simulink library "lib_fuel_converter"  (Simulink 7.9)
settings: Solver=ode45  SolverMode=SingleTasking  StartTime=0.0  StopTime=10.0  RelTol=1e-3
undefined symbols (not defined in the file or in its folder): acc_mech_eff, acc_mech_pwr, acc_mech_trq, air_cp, amb_tmp, cyc_mph, ex_gas_cp, fc_acc_mass, fc_base_mass, fc_c2i_th_cond, fc_c_init_tmp, fc_cl2h_eff, fc_CO2_to_FUELgps, fc_co_map, fc_co_map_c2h, fc_cold, fc_cold_tmp, fc_cp, fc_ct_trq, fc_eff_scale, fc_emisv, fc_exflow_map, fc_ext_sarea, fc_extmp_map, fc_fuel_den, fc_fuel_lhv, fc_fuel_map, fc_fuel_map_c2h, fc_h2x_th_cond, fc_h_air_flow, fc_h_cp, fc_h_init_tmp, fc_hc_map, fc_hc_map_c2h, fc_hood_emisv, fc_hood_sarea, fc_i2x_th_cond, fc_i_init_tmp, fc_inertia, fc_map_spd, fc_map_trq, fc_max_trq, fc_nn_model_name, fc_nox_map, fc_nox_map_c2h, fc_o2_map, fc_pm_map, fc_pm_map_c2h, fc_pwr_scale, fc_spd_scale, fc_trq_scale, fc_tstat, fc_x_init_tmp, fd_ratio, gb_num_init, gb_ratio, pow, vc_idle_spd, vc_key_on, veh_glider_mass ... (+2)
libraries: lib_fuel_converter x6, lib_etc x4
(part 2 of 4)

== system lib_fuel_converter/fuel converter  <fc> for series/spinning up or spinning down ==
  spd command (rad/s) : Inport
  engine disconnected from drivetrain : Inport  Port=2
  previous engine spd (rad/s) : Inport  Port=3
  Constant : Constant  Value=0
  Constant1 : Constant  Value=vc_idle_spd
  MinMax : MinMax  Inputs=2  SaturateOnIntegerOverflow=on  InputSameDT=on
  MinMax1 : MinMax  Function=max  Inputs=2  SaturateOnIntegerOverflow=on  InputSameDT=on
  Mux3 : Mux  Inputs=3
  Product : Product  SaturateOnIntegerOverflow=on  RndMeth=Zero  InputSameDT=on  OutDataTypeStr=Inherit: Same as first input
  Product2 : Product  SaturateOnIntegerOverflow=on  RndMeth=Zero  InputSameDT=on  OutDataTypeStr=Inherit: Same as first input
  Relational Operator : RelationalOperator  Operator=<=  InputSameDT=on
  Sum : Sum  Inputs=|++  SaturateOnIntegerOverflow=on  InputSameDT=on  OutDataTypeStr=Inherit: Same as first input
  Sum1 : Sum  Inputs=|+-  SaturateOnIntegerOverflow=on  InputSameDT=on  OutDataTypeStr=Inherit: Same as first input
  Sum2 : Sum  SaturateOnIntegerOverflow=on  InputSameDT=on  OutDataTypeStr=Inherit: Same as first input
  Switch: map torque : Switch  Threshold=eps  SaturateOnIntegerOverflow=on  InputSameDT=on
  T_closed throttle : Subsystem
  T_max : Subsystem
  alpha : Gain  Gain=1/(fc_inertia+eps)  SaturateOnIntegerOverflow=on  OutDataTypeStr=Inherit: Same as input  ParamDataTypeStr=Inherit: Same as input
  dt : Subsystem
  effect of inertia (Nm) : Subsystem
  just started spin-down/spin-up : Subsystem
  no-lag Reset Integrator : Subsystem  mask(No-lag Reset Integrator){initval=vc_idle_spd}
      mask prompts: initval "Initial Value"
      mask help: No-lag Reset Integrator
      mask Help: Integrates first input using Euler technique.\nAt the time step that input 2 <> zero,\noutput is reset to input 3.
      mask Display: disp('1/s\nw/ reset\nno lag')
  map trq (Nm) spd (rad/s) trq to drivetrain (Nm) : Outport  InitialOutput=0
  wires:
  T_max/1(T_max) -> MinMax/1
  MinMax/1 -> Switch: map torque/1
  T_closed throttle/1(T_closed throttle) -> Switch: map torque/3
  Switch: map torque/1 -> Mux3/1, Sum1/1
  Relational Operator/1 -> Switch: map torque/2
  alpha/1 -> Product/1, no-lag Reset Integrator/1(in_1)
  previous engine spd (rad/s)/1 -> T_closed throttle/1(w_APU), T_max/1(w_APU), effect of inertia (Nm)/2(prev spd), Relational Operator/1, Sum2/2
  spd command (rad/s)/1 -> Relational Operator/2, effect of inertia (Nm)/1(req'd spd (rad/s))
  no-lag Reset Integrator/1(out_1) -> MinMax1/1
  just started spin-down/spin-up/1(trigger) -> no-lag Reset Integrator/2(in_2)
  Sum2/1 -> no-lag Reset Integrator/3(in_3)
  engine disconnected from drivetrain/1 -> just started spin-down/spin-up/1(state)
  Product/1 -> Sum2/1
  dt/1(out_1) -> Product/2
  Mux3/1 -> map trq (Nm) spd (rad/s) trq to drivetrain (Nm)/1
  Constant/1 -> Mux3/3
  Constant1/1 -> Product2/1
  [engine_on] -> Product2/2
  Product2/1 -> MinMax1/2
  MinMax1/1 -> Mux3/2
  effect of inertia (Nm)/1((Nm)) -> Sum/1
  Sum/1 -> MinMax/2
  [acc_mech_trq_est] -> Sum/2
  Sum1/1 -> alpha/1
  [acc_mech_trq_est] -> Sum1/2

== system lib_fuel_converter/fuel converter  <fc> prius/Block NOTES ==
  note: This block models the internal combustion engine, and includes inertia effects,
      | performance limits, accessory loads, and temperature transient effects on fuel
      | use, engine-out emissions, and catalyst efficiency.  There are 'leads' to the
      | engine controller here, which controller determines whether the engine is on.

== system lib_fuel_converter/fuel converter  <fc> prius/fuel use and EO emis Configurable Subsystem ==
  T (Nm) : Inport
  w (rad/s) : Inport  Port=2
  fuel use and EO emis : lib_fuel_converter/configurable subsystems/fuel use and EO emis
      settings: RTWFcnNameOpts=Auto  RTWFileNameOpts=Auto
  cumulative fuel  use (gal) : Outport
  "FC ON?, EOem, MFex, Tex, O2ex" : Outport  Port=2
  Vv,Tfc : Outport  Port=3
  wires:
  T (Nm)/1 -> fuel use and EO emis/1
  w (rad/s)/1 -> fuel use and EO emis/2
  fuel use and EO emis/1 -> cumulative fuel  use (gal)/1
  fuel use and EO emis/2 -> "FC ON?, EOem, MFex, Tex, O2ex"/1
  fuel use and EO emis/3 -> Vv,Tfc/1

== system lib_fuel_converter/fuel converter  <fc> prius/providing trq (+ive or -ive) ==
  req'd trq (Nm) : Inport
  req'd spd (rad/s) : Inport  Port=2
  prev engine spd (rad/s) : Inport  Port=3
  Mux3 : Mux
  Product : Product  SaturateOnIntegerOverflow=on  RndMeth=Zero  InputSameDT=on  OutDataTypeStr=Inherit: Same as first input
  Sum1 : Sum  Inputs=+--  SaturateOnIntegerOverflow=on  InputSameDT=on  OutDataTypeStr=Inherit: Same as first input
  Sum2 : Sum  Inputs=+++  SaturateOnIntegerOverflow=on  InputSameDT=on  OutDataTypeStr=Inherit: Same as first input
  accessories (Nm) : Subsystem
  effect of inertia (Nm) : Subsystem
  enforce engine limits : Subsystem
  map trq (Nm) spd (rad/s) trq to drivetrain (Nm) accessory load (W) : Outport  InitialOutput=0
  tag scope: engine_rpm=global
  wires:
  req'd spd (rad/s)/1 -> Product/2, enforce engine limits/2(req'd engine spd (rad/s))
  Product/1 -> Mux3/4
  Sum1/1 -> Mux3/3
  Mux3/1 -> map trq (Nm) spd (rad/s) trq to drivetrain (Nm) accessory load (W)/1
  prev engine spd (rad/s)/1 -> effect of inertia (Nm)/2(prev spd)
  enforce engine limits/1(limited engine brake trq (Nm)) -> Mux3/1, Sum1/1
  enforce engine limits/2(limited engine spd (rad/s)) -> effect of inertia (Nm)/1(req'd spd (rad/s)), accessories (Nm)/1(w_APU), Mux3/2, [engine_rpm]
  req'd trq (Nm)/1 -> Sum2/1
  effect of inertia (Nm)/1((Nm)) -> Sum1/2, Sum2/2
  accessories (Nm)/1(T_acc) -> Product/1, Sum1/3, Sum2/3
  Sum2/1 -> enforce engine limits/1(req'd engine trq (Nm))

== system lib_fuel_converter/configurable subsystems/fuel use and EO emis/Block NOTES ==
  note: This block determines actual fuel use and engine-out emissions
      | given the fully hot values and the engine coolant temperature.
      | The correlations used here were developed at NREL using
      | FTP data collected under subcontract by JDM & Associates.
      | Note: PM hot/cold relation assumed same as HC

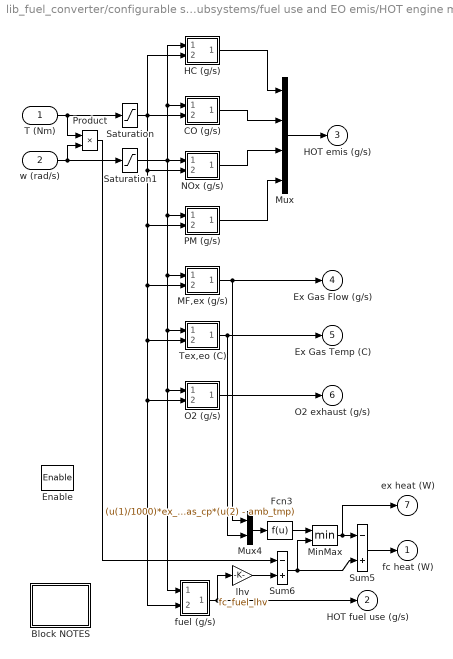
== system lib_fuel_converter/configurable subsystems/fuel use and EO emis/HOT engine maps  ==
  T (Nm) : Inport
  w (rad/s) : Inport  Port=2
  Enable : EnablePort  StatesWhenEnabling=reset
  Block NOTES : Subsystem
      mask Display: disp('Block\nNOTES')
  CO (g/s) : Subsystem  mask(2-D Table Lookup){xindex=fc_map_spd*fc_spd_scale, yindex=fc_map_trq*fc_trq_scale, table=fc_co_map*fc_spd_scale*fc_trq_scale}
      mask prompts: xindex "X Index"; yindex "Y Index"
      mask help:
      | Two Dimensional Table Lookup
      | The first input corresponds to X Index and the second input corresponds to the Y Index
      mask init:
      | sftab2chk(xindex,yindex,table);
      mask Help: This block returns a linearly interpolated intersection from the table using the X index (which corresponds to the rows of the table) and the Y index (which corresponds to the columns of the table).  Extrapolation is used.
      mask Display: plot(-10,-10,110,110,[90,50,10],[90,40,30],[90,50,10],[50,26,20],[90,50,10],[22,13,10])
  Fcn3 : Fcn  Expr=(u(1)/1000)*ex_gas_cp*(u(2) - amb_tmp)
  HC (g/s) : Subsystem  mask(2-D Table Lookup){xindex=fc_map_spd*fc_spd_scale, yindex=fc_map_trq*fc_trq_scale, table=fc_hc_map*fc_spd_scale*fc_trq_scale}
      mask prompts: xindex "X Index"; yindex "Y Index"
      mask help:
      | Two Dimensional Table Lookup
      | The first input corresponds to X Index and the second input corresponds to the Y Index
      mask init:
      | sftab2chk(xindex,yindex,table);
      mask Help: This block returns a linearly interpolated intersection from the table using the X index (which corresponds to the rows of the table) and the Y index (which corresponds to the columns of the table).  Extrapolation is used.
      mask Display: plot(-10,-10,110,110,[90,50,10],[90,40,30],[90,50,10],[50,26,20],[90,50,10],[22,13,10])
  MF,ex (g/s) : Subsystem  mask(2-D Table Lookup){xindex=fc_map_spd*fc_spd_scale, yindex=fc_map_trq*fc_trq_scale, table=fc_exflow_map*fc_spd_scale*fc_trq_scale}
      mask prompts: xindex "X Index"; yindex "Y Index"
      mask help:
      | Two Dimensional Table Lookup
      | The first input corresponds to X Index and the second input corresponds to the Y Index
      mask init:
      | sftab2chk(xindex,yindex,table);
      mask Help: This block returns a linearly interpolated intersection from the table using the X index (which corresponds to the rows of the table) and the Y index (which corresponds to the columns of the table).  Extrapolation is used.
      mask Display: plot(-10,-10,110,110,[90,50,10],[90,40,30],[90,50,10],[50,26,20],[90,50,10],[22,13,10])
  MinMax : MinMax  Inputs=2  SaturateOnIntegerOverflow=on  InputSameDT=on
  Mux : Mux
  Mux4 : Mux  Inputs=2
  NOx (g/s) : Subsystem  mask(2-D Table Lookup){xindex=fc_map_spd*fc_spd_scale, yindex=fc_map_trq*fc_trq_scale, table=fc_nox_map*fc_spd_scale*fc_trq_scale}
      mask prompts: xindex "X Index"; yindex "Y Index"
      mask help:
      | Two Dimensional Table Lookup
      | The first input corresponds to X Index and the second input corresponds to the Y Index
      mask init:
      | sftab2chk(xindex,yindex,table);
      mask Help: This block returns a linearly interpolated intersection from the table using the X index (which corresponds to the rows of the table) and the Y index (which corresponds to the columns of the table).  Extrapolation is used.
      mask Display: plot(-10,-10,110,110,[90,50,10],[90,40,30],[90,50,10],[50,26,20],[90,50,10],[22,13,10])
  O2 (g/s) : Subsystem  mask(2-D Table Lookup){xindex=fc_map_spd*fc_spd_scale, yindex=fc_map_trq*fc_trq_scale, table=fc_o2_map*fc_spd_scale*fc_trq_scale}
      mask prompts: xindex "X Index"; yindex "Y Index"
      mask help:
      | Two Dimensional Table Lookup
      | The first input corresponds to X Index and the second input corresponds to the Y Index
      mask init:
      | sftab2chk(xindex,yindex,table);
      mask Help: This block returns a linearly interpolated intersection from the table using the X index (which corresponds to the rows of the table) and the Y index (which corresponds to the columns of the table).  Extrapolation is used.
      mask Display: plot(-10,-10,110,110,[90,50,10],[90,40,30],[90,50,10],[50,26,20],[90,50,10],[22,13,10])
  PM (g/s) : Subsystem  mask(2-D Table Lookup){xindex=fc_map_spd*fc_spd_scale, yindex=fc_map_trq*fc_trq_scale, table=fc_pm_map*fc_spd_scale*fc_trq_scale}
      mask prompts: xindex "X Index"; yindex "Y Index"
      mask help:
      | Two Dimensional Table Lookup
      | The first input corresponds to X Index and the second input corresponds to the Y Index
      mask init:
      | sftab2chk(xindex,yindex,table);
      mask Help: This block returns a linearly interpolated intersection from the table using the X index (which corresponds to the rows of the table) and the Y index (which corresponds to the columns of the table).  Extrapolation is used.
      mask Display: plot(-10,-10,110,110,[90,50,10],[90,40,30],[90,50,10],[50,26,20],[90,50,10],[22,13,10])
  Product : Product  SaturateOnIntegerOverflow=on  RndMeth=Zero  InputSameDT=on  OutDataTypeStr=Inherit: Same as first input
  Saturation : Saturate  UpperLimit=max(fc_map_trq*fc_trq_scale)  LowerLimit=min(fc_map_trq*fc_trq_scale)
  Saturation1 : Saturate  UpperLimit=max(fc_map_spd*fc_spd_scale)  LowerLimit=min(fc_map_spd*fc_spd_scale)
  Sum5 : Sum  Inputs=-+  SaturateOnIntegerOverflow=on  InputSameDT=on  OutDataTypeStr=Inherit: Same as first input
  Sum6 : Sum  Inputs=-+  SaturateOnIntegerOverflow=on  InputSameDT=on  OutDataTypeStr=Inherit: Same as first input
  Tex,eo (C) : Subsystem  mask(2-D Table Lookup){xindex=fc_map_spd*fc_spd_scale, yindex=fc_map_trq*fc_trq_scale, table=fc_extmp_map}
      mask prompts: xindex "X Index"; yindex "Y Index"
      mask help:
      | Two Dimensional Table Lookup
      | The first input corresponds to X Index and the second input corresponds to the Y Index
      mask init:
      | sftab2chk(xindex,yindex,table);
      mask Help: This block returns a linearly interpolated intersection from the table using the X index (which corresponds to the rows of the table) and the Y index (which corresponds to the columns of the table).  Extrapolation is used.
      mask Display: plot(-10,-10,110,110,[90,50,10],[90,40,30],[90,50,10],[50,26,20],[90,50,10],[22,13,10])
  fuel (g/s) : Subsystem  mask(2-D Table Lookup){xindex=fc_map_spd*fc_spd_scale, yindex=fc_map_trq*fc_trq_scale, table=fc_fuel_map*fc_spd_scale*fc_trq_scale/fc_eff_scale}
      mask prompts: xindex "X Index"; yindex "Y Index"
      mask help:
      | Two Dimensional Table Lookup
      | The first input corresponds to X Index and the second input corresponds to the Y Index
      mask init:
      | sftab2chk(xindex,yindex,table);
      mask Help: This block returns a linearly interpolated intersection from the table using the X index (which corresponds to the rows of the table) and the Y index (which corresponds to the columns of the table).  Extrapolation is used.
      mask Display: plot(-10,-10,110,110,[90,50,10],[90,40,30],[90,50,10],[50,26,20],[90,50,10],[22,13,10])
  lhv : Gain  Gain=fc_fuel_lhv  SaturateOnIntegerOverflow=on  OutDataTypeStr=Inherit: Same as input  ParamDataTypeStr=Inherit: Same as input
  fc heat (W) : Outport  OutputWhenDisabled=reset  InitialOutput=eps
  HOT fuel use (g/s) : Outport  Port=2  OutputWhenDisabled=reset  InitialOutput=eps
  HOT emis (g/s) : Outport  Port=3  OutputWhenDisabled=reset  InitialOutput=eps
  Ex Gas Flow (g/s) : Outport  Port=4  OutputWhenDisabled=reset  InitialOutput=eps
  Ex Gas Temp (C) : Outport  Port=5  OutputWhenDisabled=reset  InitialOutput=amb_tmp
  O2 exhaust (g/s) : Outport  Port=6  OutputWhenDisabled=reset  InitialOutput=0
  ex heat (W) : Outport  Port=7  OutputWhenDisabled=reset  InitialOutput=eps
  wires:
  PM (g/s)/1(table out) -> Mux/4
  HC (g/s)/1(table out) -> Mux/1
  CO (g/s)/1(table out) -> Mux/2
  NOx (g/s)/1(table out) -> Mux/3
  Mux/1 -> HOT emis (g/s)/1
  MF,ex (g/s)/1(table out) -> Ex Gas Flow (g/s)/1, Mux4/1
  Tex,eo (C)/1(table out) -> Ex Gas Temp (C)/1, Mux4/2
  Saturation1/1 -> NOx (g/s)/1(x0), MF,ex (g/s)/1(x0), Tex,eo (C)/1(x0), fuel (g/s)/1(x0), O2 (g/s)/1(x0), PM (g/s)/1(x0), CO (g/s)/1(x0), HC (g/s)/1(x0)
  Saturation/1 -> CO (g/s)/2(y0), MF,ex (g/s)/2(y0), Tex,eo (C)/2(y0), fuel (g/s)/2(y0), O2 (g/s)/2(y0), PM (g/s)/2(y0), NOx (g/s)/2(y0), HC (g/s)/2(y0)
  T (Nm)/1 -> Saturation/1, Product/1
  w (rad/s)/1 -> Saturation1/1, Product/2
  Mux4/1 -> Fcn3/1
  Sum5/1 -> fc heat (W)/1
  Fcn3/1 -> MinMax/1
  MinMax/1 -> Sum5/1, ex heat (W)/1
  Sum6/1 -> Sum5/2, MinMax/2
  Product/1 -> Sum6/1
  fuel (g/s)/1(table out) -> HOT fuel use (g/s)/1, lhv/1
  lhv/1 -> Sum6/2
  O2 (g/s)/1(table out) -> O2 exhaust (g/s)/1

== system lib_fuel_converter/configurable subsystems/fuel use and EO emis/fc temp ==
  note: h
  note: x
  note: i
  note: c
  veh spd (m/s) : Inport
  key ON? : Inport  Port=2
  fc ON? : Inport  Port=3
  Qfc (W) : Inport  Port=4
  "1/ " : Gain  Gain=1/(0.2*fc_base_mass*fc_pwr_scale*fc_cp)  SaturateOnIntegerOverflow=on  OutDataTypeStr=Inherit: Same as input  ParamDataTypeStr=Inherit: Same as input
  1/Ci : Gain  Gain=1/(0.8*fc_base_mass*fc_pwr_scale*fc_cp)  SaturateOnIntegerOverflow=on  OutDataTypeStr=Inherit: Same as input  ParamDataTypeStr=Inherit: Same as input
  1/Cx : Gain  Gain=1/(fc_acc_mass*fc_pwr_scale*fc_cp)  SaturateOnIntegerOverflow=on  OutDataTypeStr=Inherit: Same as input  ParamDataTypeStr=Inherit: Same as input
  1/mcp : Gain  Gain=1/(0.1*veh_glider_mass*fc_pwr_scale*fc_h_cp)  SaturateOnIntegerOverflow=on  OutDataTypeStr=Inherit: Same as input  ParamDataTypeStr=Inherit: Same as input
  Block NOTES : Subsystem
      mask Display: disp('Block\nNOTES')
  Memory : Memory  X0=fc_h_init_tmp
  Mux3 : Mux
  Mux4 : Mux  Inputs=2
  Qc : Sum  SaturateOnIntegerOverflow=on  InputSameDT=on  OutDataTypeStr=Inherit: Same as first input
  Qc1 : Sum  Inputs=--+  SaturateOnIntegerOverflow=on  InputSameDT=on  OutDataTypeStr=Inherit: Same as first input
  Tcm : Integrator  InitialCondition=fc_c_init_tmp
  Tcx : Integrator  InitialCondition=fc_x_init_tmp
  Tcx1 : Integrator  InitialCondition=fc_i_init_tmp
  Tm : Integrator  InitialCondition=fc_h_init_tmp
  fc coolant : Subsystem  TreatAsAtomicUnit=on
  fc mass heat flow : Subsystem
  old fc coolant  temp. (C) : Subsystem
  Tfc_old  (C) : Outport  InitialOutput=0
  Qfc r,h : Outport  Port=2  InitialOutput=0
  Tfc  (C) : Outport  Port=3  InitialOutput=0
  tag scope: fc_hood_temp=global
  wires:
  Qc/1 -> "1/ "/1
  "1/ "/1 -> Tcm/1
  Qfc (W)/1 -> Qc/1
  fc mass heat flow/1(Qfc_c) -> Qc/2
  Qc1/1 -> 1/Ci/1
  1/Ci/1 -> Tcx1/1
  Tcm/1 -> Mux3/1
  fc mass heat flow/2(Qfc_i) -> Qc1/3, fc coolant/2("Qfc_i ")
  fc coolant/2(Qfc_htr) -> Qc1/2, Mux4/2
  fc coolant/1(Qfc_rad) -> Qc1/1, Mux4/1
  Tcx1/1 -> fc coolant/1(Tcl), Mux3/2
  Mux4/1 -> Qfc r,h/1
  1/Cx/1 -> Tcx/1
  fc mass heat flow/3(Qfc_x) -> 1/Cx/1
  key ON?/1 -> fc coolant/Enable
  Tcx/1 -> Mux3/3
  Tm/1 -> Mux3/4, Memory/1
  1/mcp/1 -> Tm/1
  fc mass heat flow/4(Qfc_h) -> 1/mcp/1
  Mux3/1 -> fc mass heat flow/2(fc_temp), Tfc  (C)/1
  old fc coolant  temp. (C)/1(fc coolant  temp (C)) -> Tfc_old  (C)/1
  veh spd (m/s)/1 -> old fc coolant  temp. (C)/2(veh spd), fc mass heat flow/1(veh spd)
  fc ON?/1 -> old fc coolant  temp. (C)/1(fc on?)
  Memory/1 -> [fc_hood_temp]

== system lib_fuel_converter/configurable subsystems/fuel use and EO emis/fc temp correct ==
  Coolant T (C) : Inport
  HOT fuel use (g/s) : Inport  Port=2
  HOT emis (g/s) : Inport  Port=3
  T (Nm) : Inport  Port=4
  w (rad/s) : Inport  Port=5
  Enable : EnablePort  StatesWhenEnabling=reset
  =1: use map based =0: use constant equation based : Constant  Value=fc_cold
  Switch : Switch  Threshold=eps  SaturateOnIntegerOverflow=on  InputSameDT=on
  Switch1 : Switch  Threshold=eps  SaturateOnIntegerOverflow=on  InputSameDT=on
  fc temp correct Constant Correction Factors (Equation Based) : Subsystem  TreatAsAtomicUnit=on
  fc temp correct Variable Correction Factors (Map Based) : Subsystem  TreatAsAtomicUnit=on
  fc_cold=0 : Logic  Operator=NOT
  fuel use (g/s) : Outport  OutputWhenDisabled=reset  InitialOutput=0
  EO emis (g/s) : Outport  Port=2  OutputWhenDisabled=reset  InitialOutput=0
  wires:
  =1: use map based =0: use constant equation based/1 -> fc_cold=0/1, fc temp correct Variable Correction Factors (Map Based)/Enable
  Coolant T (C)/1 -> fc temp correct Constant Correction Factors (Equation Based)/1(Coolant T (C)), fc temp correct Variable Correction Factors (Map Based)/1(Coolant T (C))
  HOT fuel use (g/s)/1 -> fc temp correct Constant Correction Factors (Equation Based)/2(HOT fuel use (g/s)), fc temp correct Variable Correction Factors (Map Based)/2(HOT fuel use (g/s))
  HOT emis (g/s)/1 -> fc temp correct Constant Correction Factors (Equation Based)/3(HOT emis (g/s)), fc temp correct Variable Correction Factors (Map Based)/3(HOT emis (g/s))
  fc temp correct Constant Correction Factors (Equation Based)/1(fuel use (g/s)) -> Switch/1
  fc_cold=0/1 -> fc temp correct Constant Correction Factors (Equation Based)/Enable, Switch/2, Switch1/2
  fc temp correct Variable Correction Factors (Map Based)/1(fuel use (g/s)) -> Switch/3
  fc temp correct Constant Correction Factors (Equation Based)/2(EO emis (g/s)) -> Switch1/1
  fc temp correct Variable Correction Factors (Map Based)/2(EO emis (g/s)) -> Switch1/3
  Switch/1 -> fuel use (g/s)/1
  Switch1/1 -> EO emis (g/s)/1
  T (Nm)/1 -> fc temp correct Variable Correction Factors (Map Based)/4(T (Nm))
  w (rad/s)/1 -> fc temp correct Variable Correction Factors (Map Based)/5(w (rad/s))

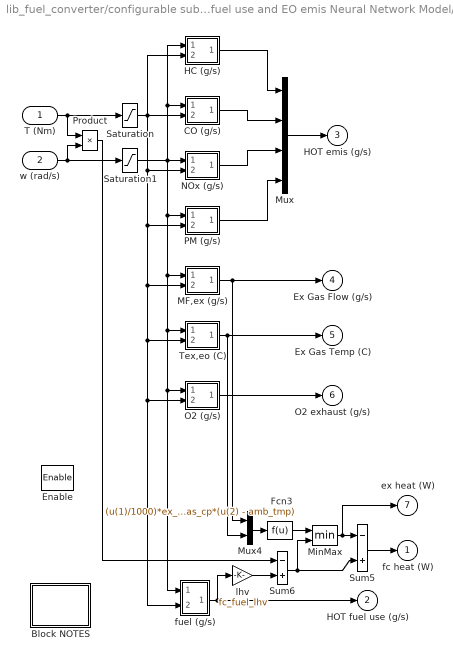
== system lib_fuel_converter/configurable subsystems/fuel use and EO emis Neural Network Model/HOT engine maps  ==
  T (Nm) : Inport
  w (rad/s) : Inport  Port=2
  Enable : EnablePort  StatesWhenEnabling=reset
  Block NOTES : Subsystem
      mask Display: disp('Block\nNOTES')
  CO (g/s) : Subsystem  mask(2-D Table Lookup){xindex=fc_map_spd*fc_spd_scale, yindex=fc_map_trq*fc_trq_scale, table=fc_co_map*fc_spd_scale*fc_trq_scale}
      mask prompts: xindex "X Index"; yindex "Y Index"
      mask help:
      | Two Dimensional Table Lookup
      | The first input corresponds to X Index and the second input corresponds to the Y Index
      mask init:
      | sftab2chk(xindex,yindex,table);
      mask Help: This block returns a linearly interpolated intersection from the table using the X index (which corresponds to the rows of the table) and the Y index (which corresponds to the columns of the table).  Extrapolation is used.
      mask Display: plot(-10,-10,110,110,[90,50,10],[90,40,30],[90,50,10],[50,26,20],[90,50,10],[22,13,10])
  Fcn3 : Fcn  Expr=(u(1)/1000)*ex_gas_cp*(u(2) - amb_tmp)
  HC (g/s) : Subsystem  mask(2-D Table Lookup){xindex=fc_map_spd*fc_spd_scale, yindex=fc_map_trq*fc_trq_scale, table=fc_hc_map*fc_spd_scale*fc_trq_scale}
      mask prompts: xindex "X Index"; yindex "Y Index"
      mask help:
      | Two Dimensional Table Lookup
      | The first input corresponds to X Index and the second input corresponds to the Y Index
      mask init:
      | sftab2chk(xindex,yindex,table);
      mask Help: This block returns a linearly interpolated intersection from the table using the X index (which corresponds to the rows of the table) and the Y index (which corresponds to the columns of the table).  Extrapolation is used.
      mask Display: plot(-10,-10,110,110,[90,50,10],[90,40,30],[90,50,10],[50,26,20],[90,50,10],[22,13,10])
  MF,ex (g/s) : Subsystem  mask(2-D Table Lookup){xindex=fc_map_spd*fc_spd_scale, yindex=fc_map_trq*fc_trq_scale, table=fc_exflow_map*fc_spd_scale*fc_trq_scale}
      mask prompts: xindex "X Index"; yindex "Y Index"
      mask help:
      | Two Dimensional Table Lookup
      | The first input corresponds to X Index and the second input corresponds to the Y Index
      mask init:
      | sftab2chk(xindex,yindex,table);
      mask Help: This block returns a linearly interpolated intersection from the table using the X index (which corresponds to the rows of the table) and the Y index (which corresponds to the columns of the table).  Extrapolation is used.
      mask Display: plot(-10,-10,110,110,[90,50,10],[90,40,30],[90,50,10],[50,26,20],[90,50,10],[22,13,10])
  MinMax : MinMax  Inputs=2  SaturateOnIntegerOverflow=on  InputSameDT=on
  Mux : Mux
  Mux4 : Mux  Inputs=2
  NOx (g/s) : Subsystem  mask(2-D Table Lookup){xindex=fc_map_spd*fc_spd_scale, yindex=fc_map_trq*fc_trq_scale, table=fc_nox_map*fc_spd_scale*fc_trq_scale}
      mask prompts: xindex "X Index"; yindex "Y Index"
      mask help:
      | Two Dimensional Table Lookup
      | The first input corresponds to X Index and the second input corresponds to the Y Index
      mask init:
      | sftab2chk(xindex,yindex,table);
      mask Help: This block returns a linearly interpolated intersection from the table using the X index (which corresponds to the rows of the table) and the Y index (which corresponds to the columns of the table).  Extrapolation is used.
      mask Display: plot(-10,-10,110,110,[90,50,10],[90,40,30],[90,50,10],[50,26,20],[90,50,10],[22,13,10])
  O2 (g/s) : Subsystem  mask(2-D Table Lookup){xindex=fc_map_spd*fc_spd_scale, yindex=fc_map_trq*fc_trq_scale, table=fc_o2_map*fc_spd_scale*fc_trq_scale}
      mask prompts: xindex "X Index"; yindex "Y Index"
      mask help:
      | Two Dimensional Table Lookup
      | The first input corresponds to X Index and the second input corresponds to the Y Index
      mask init:
      | sftab2chk(xindex,yindex,table);
      mask Help: This block returns a linearly interpolated intersection from the table using the X index (which corresponds to the rows of the table) and the Y index (which corresponds to the columns of the table).  Extrapolation is used.
      mask Display: plot(-10,-10,110,110,[90,50,10],[90,40,30],[90,50,10],[50,26,20],[90,50,10],[22,13,10])
  PM (g/s) : Subsystem  mask(2-D Table Lookup){xindex=fc_map_spd*fc_spd_scale, yindex=fc_map_trq*fc_trq_scale, table=fc_pm_map*fc_spd_scale*fc_trq_scale}
      mask prompts: xindex "X Index"; yindex "Y Index"
      mask help:
      | Two Dimensional Table Lookup
      | The first input corresponds to X Index and the second input corresponds to the Y Index
      mask init:
      | sftab2chk(xindex,yindex,table);
      mask Help: This block returns a linearly interpolated intersection from the table using the X index (which corresponds to the rows of the table) and the Y index (which corresponds to the columns of the table).  Extrapolation is used.
      mask Display: plot(-10,-10,110,110,[90,50,10],[90,40,30],[90,50,10],[50,26,20],[90,50,10],[22,13,10])
  Product : Product  SaturateOnIntegerOverflow=on  RndMeth=Zero  InputSameDT=on  OutDataTypeStr=Inherit: Same as first input
  Saturation : Saturate  UpperLimit=max(fc_map_trq*fc_trq_scale)  LowerLimit=min(fc_map_trq*fc_trq_scale)
  Saturation1 : Saturate  UpperLimit=max(fc_map_spd*fc_spd_scale)  LowerLimit=min(fc_map_spd*fc_spd_scale)
  Sum5 : Sum  Inputs=-+  SaturateOnIntegerOverflow=on  InputSameDT=on  OutDataTypeStr=Inherit: Same as first input
  Sum6 : Sum  Inputs=-+  SaturateOnIntegerOverflow=on  InputSameDT=on  OutDataTypeStr=Inherit: Same as first input
  Tex,eo (C) : Subsystem  mask(2-D Table Lookup){xindex=fc_map_spd*fc_spd_scale, yindex=fc_map_trq*fc_trq_scale, table=fc_extmp_map}
      mask prompts: xindex "X Index"; yindex "Y Index"
      mask help:
      | Two Dimensional Table Lookup
      | The first input corresponds to X Index and the second input corresponds to the Y Index
      mask init:
      | sftab2chk(xindex,yindex,table);
      mask Help: This block returns a linearly interpolated intersection from the table using the X index (which corresponds to the rows of the table) and the Y index (which corresponds to the columns of the table).  Extrapolation is used.
      mask Display: plot(-10,-10,110,110,[90,50,10],[90,40,30],[90,50,10],[50,26,20],[90,50,10],[22,13,10])
  fuel (g/s) : Subsystem  mask(2-D Table Lookup){xindex=fc_map_spd*fc_spd_scale, yindex=fc_map_trq*fc_trq_scale, table=fc_fuel_map*fc_spd_scale*fc_trq_scale/fc_eff_scale}
      mask prompts: xindex "X Index"; yindex "Y Index"
      mask help:
      | Two Dimensional Table Lookup
      | The first input corresponds to X Index and the second input corresponds to the Y Index
      mask init:
      | sftab2chk(xindex,yindex,table);
      mask Help: This block returns a linearly interpolated intersection from the table using the X index (which corresponds to the rows of the table) and the Y index (which corresponds to the columns of the table).  Extrapolation is used.
      mask Display: plot(-10,-10,110,110,[90,50,10],[90,40,30],[90,50,10],[50,26,20],[90,50,10],[22,13,10])
  lhv : Gain  Gain=fc_fuel_lhv  SaturateOnIntegerOverflow=on  OutDataTypeStr=Inherit: Same as input  ParamDataTypeStr=Inherit: Same as input
  fc heat (W) : Outport  OutputWhenDisabled=reset  InitialOutput=eps
  HOT fuel use (g/s) : Outport  Port=2  OutputWhenDisabled=reset  InitialOutput=eps
  HOT emis (g/s) : Outport  Port=3  OutputWhenDisabled=reset  InitialOutput=eps
  Ex Gas Flow (g/s) : Outport  Port=4  OutputWhenDisabled=reset  InitialOutput=eps
  Ex Gas Temp (C) : Outport  Port=5  OutputWhenDisabled=reset  InitialOutput=amb_tmp
  O2 exhaust (g/s) : Outport  Port=6  OutputWhenDisabled=reset  InitialOutput=0
  ex heat (W) : Outport  Port=7  OutputWhenDisabled=reset  InitialOutput=eps
  wires:
  O2 (g/s)/1(table out) -> O2 exhaust (g/s)/1
  lhv/1 -> Sum6/2
  fuel (g/s)/1(table out) -> lhv/1, HOT fuel use (g/s)/1
  Product/1 -> Sum6/1
  Sum6/1 -> MinMax/2, Sum5/2
  MinMax/1 -> ex heat (W)/1, Sum5/1
  Fcn3/1 -> MinMax/1
  Sum5/1 -> fc heat (W)/1
  Mux4/1 -> Fcn3/1
  w (rad/s)/1 -> Product/2, Saturation1/1
  T (Nm)/1 -> Product/1, Saturation/1
  Saturation/1 -> HC (g/s)/2(y0), CO (g/s)/2(y0), O2 (g/s)/2(y0), fuel (g/s)/2(y0), Tex,eo (C)/2(y0), MF,ex (g/s)/2(y0), PM (g/s)/2(y0), NOx (g/s)/2(y0)
  Saturation1/1 -> HC (g/s)/1(x0), CO (g/s)/1(x0), O2 (g/s)/1(x0), fuel (g/s)/1(x0), Tex,eo (C)/1(x0), MF,ex (g/s)/1(x0), PM (g/s)/1(x0), NOx (g/s)/1(x0)
  Tex,eo (C)/1(table out) -> Mux4/2, Ex Gas Temp (C)/1
  MF,ex (g/s)/1(table out) -> Mux4/1, Ex Gas Flow (g/s)/1
  Mux/1 -> HOT emis (g/s)/1
  NOx (g/s)/1(table out) -> Mux/3
  CO (g/s)/1(table out) -> Mux/2
  HC (g/s)/1(table out) -> Mux/1
  PM (g/s)/1(table out) -> Mux/4

== system lib_fuel_converter/configurable subsystems/fuel use and EO emis Neural Network Model/fc temp ==
  note: c
  note: i
  note: x
  note: h
  veh spd (m/s) : Inport
  key ON? : Inport  Port=2
  fc ON? : Inport  Port=3
  Qfc (W) : Inport  Port=4
  "1/ " : Gain  Gain=1/(0.2*fc_base_mass*fc_pwr_scale*fc_cp)  SaturateOnIntegerOverflow=on  OutDataTypeStr=Inherit: Same as input  ParamDataTypeStr=Inherit: Same as input
  1/Ci : Gain  Gain=1/(0.8*fc_base_mass*fc_pwr_scale*fc_cp)  SaturateOnIntegerOverflow=on  OutDataTypeStr=Inherit: Same as input  ParamDataTypeStr=Inherit: Same as input
  1/Cx : Gain  Gain=1/(fc_acc_mass*fc_pwr_scale*fc_cp)  SaturateOnIntegerOverflow=on  OutDataTypeStr=Inherit: Same as input  ParamDataTypeStr=Inherit: Same as input
  1/mcp : Gain  Gain=1/(0.1*veh_glider_mass*fc_pwr_scale*fc_h_cp)  SaturateOnIntegerOverflow=on  OutDataTypeStr=Inherit: Same as input  ParamDataTypeStr=Inherit: Same as input
  Block NOTES : Subsystem
      mask Display: disp('Block\nNOTES')
  Mux3 : Mux
  Mux4 : Mux  Inputs=2
  Qc : Sum  SaturateOnIntegerOverflow=on  InputSameDT=on  OutDataTypeStr=Inherit: Same as first input
  Qc1 : Sum  Inputs=--+  SaturateOnIntegerOverflow=on  InputSameDT=on  OutDataTypeStr=Inherit: Same as first input
  Tcm : Integrator  InitialCondition=fc_c_init_tmp
  Tcx : Integrator  InitialCondition=fc_x_init_tmp
  Tcx1 : Integrator  InitialCondition=fc_i_init_tmp
  Tm : Integrator  InitialCondition=fc_h_init_tmp
  fc coolant : Subsystem  TreatAsAtomicUnit=on
  fc mass heat flow : Subsystem
  old fc coolant  temp. (C) : Subsystem
  Tfc_old  (C) : Outport  InitialOutput=0
  Qfc r,h : Outport  Port=2  InitialOutput=0
  Tfc  (C) : Outport  Port=3  InitialOutput=0
  wires:
  fc ON?/1 -> old fc coolant  temp. (C)/1(fc on?)
  veh spd (m/s)/1 -> fc mass heat flow/1(veh spd), old fc coolant  temp. (C)/2(veh spd)
  old fc coolant  temp. (C)/1(fc coolant  temp (C)) -> Tfc_old  (C)/1
  Mux3/1 -> Tfc  (C)/1, fc mass heat flow/2(fc_temp)
  fc mass heat flow/4(Qfc_h) -> 1/mcp/1
  1/mcp/1 -> Tm/1
  Tm/1 -> Mux3/4
  Tcx/1 -> Mux3/3
  key ON?/1 -> fc coolant/Enable
  fc mass heat flow/3(Qfc_x) -> 1/Cx/1
  1/Cx/1 -> Tcx/1
  Mux4/1 -> Qfc r,h/1
  Tcx1/1 -> Mux3/2, fc coolant/1(Tcl)
  fc coolant/1(Qfc_rad) -> Mux4/1, Qc1/1
  fc coolant/2(Qfc_htr) -> Mux4/2, Qc1/2
  fc mass heat flow/2(Qfc_i) -> fc coolant/2("Qfc_i "), Qc1/3
  Tcm/1 -> Mux3/1
  1/Ci/1 -> Tcx1/1
  Qc1/1 -> 1/Ci/1
  fc mass heat flow/1(Qfc_c) -> Qc/2
  Qfc (W)/1 -> Qc/1
  "1/ "/1 -> Tcm/1
  Qc/1 -> "1/ "/1

== system lib_fuel_converter/configurable subsystems/fuel use and EO emis Neural Network Model/fc temp correct ==
  Coolant T (C) : Inport
  HOT fuel use (g/s) : Inport  Port=2
  HOT emis (g/s) : Inport  Port=3
  T (Nm) : Inport  Port=4
  w (rad/s) : Inport  Port=5
  Enable : EnablePort  StatesWhenEnabling=reset
  =1: use map based =0: use constant equation based : Constant  Value=fc_cold
  Switch : Switch  Threshold=eps  SaturateOnIntegerOverflow=on  InputSameDT=on
  Switch1 : Switch  Threshold=eps  SaturateOnIntegerOverflow=on  InputSameDT=on
  fc temp correct Constant Correction Factors (Equation Based) : Subsystem  TreatAsAtomicUnit=on
  fc temp correct Variable Correction Factors (Map Based) : Subsystem  TreatAsAtomicUnit=on
  fc_cold=0 : Logic  Operator=NOT
  fuel use (g/s) : Outport  OutputWhenDisabled=reset  InitialOutput=0
  EO emis (g/s) : Outport  Port=2  OutputWhenDisabled=reset  InitialOutput=0
  wires:
  w (rad/s)/1 -> fc temp correct Variable Correction Factors (Map Based)/5(w (rad/s))
  T (Nm)/1 -> fc temp correct Variable Correction Factors (Map Based)/4(T (Nm))
  Switch1/1 -> EO emis (g/s)/1
  Switch/1 -> fuel use (g/s)/1
  fc temp correct Variable Correction Factors (Map Based)/2(EO emis (g/s)) -> Switch1/3
  fc temp correct Constant Correction Factors (Equation Based)/2(EO emis (g/s)) -> Switch1/1
  fc temp correct Variable Correction Factors (Map Based)/1(fuel use (g/s)) -> Switch/3
  fc_cold=0/1 -> Switch1/2, Switch/2, fc temp correct Constant Correction Factors (Equation Based)/Enable
  fc temp correct Constant Correction Factors (Equation Based)/1(fuel use (g/s)) -> Switch/1
  HOT emis (g/s)/1 -> fc temp correct Variable Correction Factors (Map Based)/3(HOT emis (g/s)), fc temp correct Constant Correction Factors (Equation Based)/3(HOT emis (g/s))
  HOT fuel use (g/s)/1 -> fc temp correct Variable Correction Factors (Map Based)/2(HOT fuel use (g/s)), fc temp correct Constant Correction Factors (Equation Based)/2(HOT fuel use (g/s))
  Coolant T (C)/1 -> fc temp correct Variable Correction Factors (Map Based)/1(Coolant T (C)), fc temp correct Constant Correction Factors (Equation Based)/1(Coolant T (C))
  =1: use map based =0: use constant equation based/1 -> fc temp correct Variable Correction Factors (Map Based)/Enable, fc_cold=0/1

== system lib_fuel_converter/configurable subsystems/fuel use and EO emis Neural Network Model/nn thermal calcs ==
  gpsCO2 : Inport
  pwr (W) : Inport  Port=2
  ex gas flow (g/s) : Inport  Port=3
  ex gas tmp : Inport  Port=4
  (g/s CO2) to (g/s fuel) : Gain  Gain=fc_CO2_to_FUELgps  SaturateOnIntegerOverflow=on  OutDataTypeStr=Inherit: Same as input  ParamDataTypeStr=Inherit: Same as input
  Fcn3 : Fcn  Expr=(u(1)/1000)*ex_gas_cp*(u(2) - amb_tmp)
  MinMax : MinMax  Inputs=2  SaturateOnIntegerOverflow=on  InputSameDT=on
  Mux4 : Mux  Inputs=2
  Sum5 : Sum  Inputs=-+  SaturateOnIntegerOverflow=on  InputSameDT=on  OutDataTypeStr=Inherit: Same as first input
  Sum6 : Sum  Inputs=-+  SaturateOnIntegerOverflow=on  InputSameDT=on  OutDataTypeStr=Inherit: Same as first input
  lhv : Gain  Gain=fc_fuel_lhv  SaturateOnIntegerOverflow=on  OutDataTypeStr=Inherit: Same as input  ParamDataTypeStr=Inherit: Same as input
  fc heat (W) : Outport  OutputWhenDisabled=reset  InitialOutput=eps
  HOT fuel use (g/s) : Outport  Port=2  OutputWhenDisabled=reset  InitialOutput=eps
  ex heat (W) : Outport  Port=3  OutputWhenDisabled=reset  InitialOutput=eps
  wires:
  lhv/1 -> Sum6/2
  [fuel_gps] -> lhv/1, HOT fuel use (g/s)/1
  Sum6/1 -> MinMax/2, Sum5/2
  MinMax/1 -> ex heat (W)/1, Sum5/1
  Fcn3/1 -> MinMax/1
  Sum5/1 -> fc heat (W)/1
  Mux4/1 -> Fcn3/1
  gpsCO2/1 -> (g/s CO2) to (g/s fuel)/1
  (g/s CO2) to (g/s fuel)/1 -> [fuel_gps]
  pwr (W)/1 -> Sum6/1
  ex gas tmp/1 -> Mux4/2
  ex gas flow (g/s)/1 -> Mux4/1

== system lib_fuel_converter/fuel converter  <fc>/engine speed estimator/Block NOTES ==
  note: If the clutch is engaged and the trace was missed in the previous time step:
      | The estimated engine speed for the current time step is the actual engine
      | speed from the previous time step.
      |
      | If the clutch is disengaged and the speed is commanded to increase (spin up):
      | The engine speed is the lesser of the commanded speed and the maximum
      | speed attainable given the engine capability.
      |
      | If the clutch is disengaged at the speed is commanded to decrease (spin down):
      | The engine speed is computed by integrating with respect to time the ratio of
      |  closed-throttle torque to engine inertia.
      |
      | Otherwise:
      | The engine speed is equal to the speed command, but no greater than the
      | engine's maximum speed nor less than the engine's idle speed (if the engine is on.)

== system lib_fuel_converter/fuel converter  <fc>/engine speed estimator/dt ==
  Clock : Clock
  Memory1 : Memory  X0=-0.1
  Sum1 : Sum  Inputs=+-  SaturateOnIntegerOverflow=on  InputSameDT=on  OutDataTypeStr=Inherit: Same as first input
  out_1 : Outport  InitialOutput=0
  wires:
  Clock/1 -> Sum1/1, Memory1/1
  Memory1/1 -> Sum1/2
  Sum1/1 -> out_1/1

== system lib_fuel_converter/fuel converter  <fc>/engine speed estimator/effect of inertia (Nm) ==
  req'd spd (rad/s) : Inport
  prev spd : Inport  Port=2
  Clock : Clock
  Constant : Constant  Value=fc_inertia
  Memory : Memory  X0=-0.1
  Product1 : Product  Inputs=**/  SaturateOnIntegerOverflow=on  RndMeth=Zero  InputSameDT=on  OutDataTypeStr=Inherit: Same as first input
  Sum : Sum  Inputs=+-  SaturateOnIntegerOverflow=on  InputSameDT=on  OutDataTypeStr=Inherit: Same as first input
  Sum1 : Sum  Inputs=+-  SaturateOnIntegerOverflow=on  InputSameDT=on  OutDataTypeStr=Inherit: Same as first input
  (Nm) : Outport  InitialOutput=0
  wires:
  Sum/1 -> Product1/2
  Sum1/1 -> Product1/3
  req'd spd (rad/s)/1 -> Sum/1
  prev spd/1 -> Sum/2
  Product1/1 -> (Nm)/1
  Memory/1 -> Sum1/2
  Clock/1 -> Memory/1, Sum1/1
  Constant/1 -> Product1/1

== system lib_fuel_converter/fuel converter  <fc>/engine speed estimator/just started spin-down/spin-up ==
  state : Inport
  Logical Operator : Logic
  Logical Operator1 : Logic  Operator=NOT  Inputs=1
  Memory1 : Memory  X0=1
  trigger : Outport  InitialOutput=0
  wires:
  Memory1/1 -> Logical Operator1/1
  Logical Operator1/1 -> Logical Operator/2
  Logical Operator/1 -> trigger/1
  state/1 -> Logical Operator/1, Memory1/1

== system lib_fuel_converter/fuel converter  <fc>/engine speed estimator/no-lag Reset Integrator ==
  in_1 : Inport
  in_2 : Inport  Port=2
  in_3 : Inport  Port=3
  Constant : Constant  Value=0
  Memory : Memory  X0=initval
  Product : Product  SaturateOnIntegerOverflow=on  RndMeth=Zero  InputSameDT=on  OutDataTypeStr=Inherit: Same as first input
  Sum : Sum  SaturateOnIntegerOverflow=on  InputSameDT=on  OutDataTypeStr=Inherit: Same as first input
  Switch : Switch  Threshold=eps  SaturateOnIntegerOverflow=on  InputSameDT=on
  dt : Subsystem
  in_2==0 : RelationalOperator  Operator===  InputSameDT=on
  out_1 : Outport  InitialOutput=0
  wires:
  in_3/1 -> Switch/3
  in_2/1 -> in_2==0/1
  in_1/1 -> Product/2
  dt/1(out_1) -> Product/1
  Product/1 -> Sum/2
  Memory/1 -> Sum/1
  Sum/1 -> Switch/1
  Switch/1 -> out_1/1, Memory/1
  in_2==0/1 -> Switch/2
  Constant/1 -> in_2==0/2

== system lib_fuel_converter/fuel converter  <fc>/engine torque/Block NOTES ==
  note: If the engine is not spinning down with the clutch disengaged:
      | 1.  Engine brake (aka map) torque is given by the required shaft
      | torque plus enough torque to accelerate the engine's rotating
      | parts as commanded and torque to power the accessories,
      | subject to the engine's torque limits at the current speed.
      | 2.  Shaft torque is engine brake torque less the effects of inertia
      | and accessories.
      |
      | If the engine is spinning down:
      | 1.  Engine brake/map torque is the closed-throttle torque.
      | 2.  Shaft torque is zero.

== system lib_fuel_converter/fuel converter  <fc>/engine torque/T_closed throttle ==
  w_APU : Inport
  Saturation : Saturate  UpperLimit=max(fc_map_spd)*fc_spd_scale  LowerLimit=min(fc_map_spd)*fc_spd_scale
  ctt lookup : Lookup  InputValues=fc_map_spd*fc_spd_scale  Table=fc_ct_trq*fc_trq_scale  SaturateOnIntegerOverflow=on
  T_closed throttle : Outport  InitialOutput=0
  wires:
  ctt lookup/1 -> T_closed throttle/1
  Saturation/1 -> ctt lookup/1
  w_APU/1 -> Saturation/1

== system lib_fuel_converter/fuel converter  <fc>/engine torque/T_max ==
  w_APU : Inport
  Saturation1 : Saturate  UpperLimit=max(fc_map_spd)*fc_spd_scale  LowerLimit=min(fc_map_spd)*fc_spd_scale
  max_torque lookup : Lookup  InputValues=fc_map_spd*fc_spd_scale  Table=fc_max_trq*fc_trq_scale  SaturateOnIntegerOverflow=on
  T_max : Outport  InitialOutput=0
  tag scope: engine_rpm=global
  wires:
  w_APU/1 -> Saturation1/1
  max_torque lookup/1 -> T_max/1
  Saturation1/1 -> max_torque lookup/1, [engine_rpm]

== system lib_fuel_converter/fuel converter  <fc>/engine torque/effect of inertia (Nm) ==
  engine spd (rad/s) : Inport
  >=0 : Saturate  UpperLimit=inf  LowerLimit=0
  Block NOTES : Subsystem
      mask Display: disp('Block\nNOTES')
  Clock : Clock
  Constant : Constant  Value=fc_inertia
  Constant1 : Constant  Value=max(fc_max_trq)*fc_trq_scale
  Constant2 : Constant  Value=0.01
  Memory : Memory  X0=-0.1
  Memory1 : Memory  X0=vc_idle_spd*vc_key_on(1,2)
  Memory2 : Memory
  MinMax : MinMax  Inputs=2  SaturateOnIntegerOverflow=on  InputSameDT=on
  Product : Product  SaturateOnIntegerOverflow=on  RndMeth=Zero  InputSameDT=on  OutDataTypeStr=Inherit: Same as first input
  Product1 : Product  Inputs=*/*  SaturateOnIntegerOverflow=on  RndMeth=Zero  InputSameDT=on  OutDataTypeStr=Inherit: Same as first input
  Relational : RelationalOperator  Operator=>  InputSameDT=on
  Sum : Sum  Inputs=+-  SaturateOnIntegerOverflow=on  InputSameDT=on  OutDataTypeStr=Inherit: Same as first input
  Sum1 : Sum  Inputs=+-  SaturateOnIntegerOverflow=on  InputSameDT=on  OutDataTypeStr=Inherit: Same as first input
  Sum2 : Sum  Inputs=-+  SaturateOnIntegerOverflow=on  InputSameDT=on  OutDataTypeStr=Inherit: Same as first input
  Switch : Switch  Threshold=eps  SaturateOnIntegerOverflow=on  InputSameDT=on
  engine inertia as a function of total vehicle inertia (generous approximation) : lib_fuel_converter/Submodel/engine inertia as a function of total vehicle inertia (generous approximation)
      settings: RTWFcnNameOpts=Auto  RTWFileNameOpts=Auto
  (Nm) : Outport  InitialOutput=0
  wires:
  Sum/1 -> >=0/1, Switch/3
  Memory1/1 -> Sum/2
  Product/1 -> MinMax/1
  Constant1/1 -> Product/2
  engine inertia as a function of total vehicle inertia (generous approximation)/1 -> Product/1
  Product1/1 -> MinMax/2
  MinMax/1 -> (Nm)/1
  [cyc_mph_r] -> Sum2/2
  [mpha] -> Sum2/1
  Switch/1 -> Product1/1
  Sum1/1 -> Product1/2
  Constant/1 -> Product1/3
  Memory/1 -> Sum1/2
  Clock/1 -> Memory/1, Sum1/1
  Memory2/1 -> Switch/2
  Relational/1 -> Memory2/1
  >=0/1 -> Switch/1
  Sum2/1 -> Relational/1
  Constant2/1 -> Relational/2
  engine spd (rad/s)/1 -> Memory1/1, Sum/1

== system lib_fuel_converter/fuel converter  <fc> for series/providing trq (+ive or -ive)/effect of inertia (Nm) ==
  note: if initial speed is >0 and it is the
      | first time step ignore inertial loads
      | tm:2/6/01
  req'd spd (rad/s) : Inport
  prev spd : Inport  Port=2
  Clock : Clock
  Constant : Constant  Value=fc_inertia
  Constant1 : Constant  Value=cyc_mph(1,2)
  Logical Operator : Logic  Operator=NAND
  Logical Operator1 : Logic  Operator=NOT
  Memory : Memory  X0=-0.1
  Memory1 : Memory
  Product1 : Product  Inputs=**/*  SaturateOnIntegerOverflow=on  RndMeth=Zero  InputSameDT=on  OutDataTypeStr=Inherit: Same as first input
  Sum : Sum  Inputs=+-  SaturateOnIntegerOverflow=on  InputSameDT=on  OutDataTypeStr=Inherit: Same as first input
  Sum1 : Sum  Inputs=+-  SaturateOnIntegerOverflow=on  InputSameDT=on  OutDataTypeStr=Inherit: Same as first input
  (Nm) : Outport  InitialOutput=0
  wires:
  Constant/1 -> Product1/1
  Clock/1 -> Sum1/1, Memory/1, Memory1/1
  Memory/1 -> Sum1/2
  Product1/1 -> (Nm)/1
  prev spd/1 -> Sum/2
  req'd spd (rad/s)/1 -> Sum/1
  Sum1/1 -> Product1/3
  Sum/1 -> Product1/2
  Logical Operator/1 -> Product1/4
  Constant1/1 -> Logical Operator/1
  Memory1/1 -> Logical Operator1/1
  Logical Operator1/1 -> Logical Operator/2

== system lib_fuel_converter/fuel converter  <fc> for series/providing trq (+ive or -ive)/enforce engine limits ==
  req'd engine trq (Nm) : Inport
  req'd engine spd (rad/s) : Inport  Port=2
  Block NOTES : Subsystem
      mask Display: disp('Block\nNOTES')
  MinMax : MinMax  Inputs=2  SaturateOnIntegerOverflow=on  InputSameDT=on
  MinMax1 : MinMax  Function=max  Inputs=2  SaturateOnIntegerOverflow=on  InputSameDT=on
  Relational Operator : RelationalOperator  Operator=~=  InputSameDT=on
  Saturation : Saturate  UpperLimit=max(fc_map_spd)*fc_spd_scale  LowerLimit=0
  T_closed throttle : Subsystem
  T_max : Subsystem
  clutch disengaged1 : RelationalOperator  Operator=~=  InputSameDT=on
  limited engine brake trq (Nm) : Outport
  limited engine spd (rad/s) : Outport  Port=2
  tag scope: fc_spd_limited=global, fc_trq_limited=global
  wires:
  T_closed throttle/1(T_closed throttle) -> MinMax1/2
  req'd engine spd (rad/s)/1 -> Relational Operator/1, Saturation/1
  Saturation/1 -> Relational Operator/2, limited engine spd (rad/s)/1, T_max/1(w_APU), T_closed throttle/1(w_APU)
  req'd engine trq (Nm)/1 -> clutch disengaged1/1, MinMax/1
  MinMax1/1 -> clutch disengaged1/2, limited engine brake trq (Nm)/1
  clutch disengaged1/1 -> [fc_trq_limited]
  T_max/1(T_max) -> MinMax/2
  MinMax/1 -> MinMax1/1
  Relational Operator/1 -> [fc_spd_limited]

== system lib_fuel_converter/fuel converter  <fc> for series/spinning up or spinning down/T_closed throttle ==
  w_APU : Inport
  Saturation : Saturate  UpperLimit=max(fc_map_spd)*fc_spd_scale  LowerLimit=min(fc_map_spd)*fc_spd_scale
  ctt lookup : Lookup  InputValues=fc_map_spd*fc_spd_scale  Table=fc_ct_trq*fc_trq_scale  SaturateOnIntegerOverflow=on
  T_closed throttle : Outport  InitialOutput=0
  wires:
  ctt lookup/1 -> T_closed throttle/1
  Saturation/1 -> ctt lookup/1
  w_APU/1 -> Saturation/1

== system lib_fuel_converter/fuel converter  <fc> for series/spinning up or spinning down/T_max ==
  w_APU : Inport
  Saturation1 : Saturate  UpperLimit=max(fc_map_spd)*fc_spd_scale  LowerLimit=min(fc_map_spd)*fc_spd_scale
  max_torque lookup : Lookup  InputValues=fc_map_spd*fc_spd_scale  Table=fc_max_trq*fc_trq_scale  SaturateOnIntegerOverflow=on
  T_max : Outport  InitialOutput=0
  wires:
  Saturation1/1 -> max_torque lookup/1
  w_APU/1 -> Saturation1/1
  max_torque lookup/1 -> T_max/1

== system lib_fuel_converter/fuel converter  <fc> for series/spinning up or spinning down/dt ==
  Clock : Clock
  Memory1 : Memory  X0=-0.1
  Sum1 : Sum  Inputs=+-  SaturateOnIntegerOverflow=on  InputSameDT=on  OutDataTypeStr=Inherit: Same as first input
  out_1 : Outport  InitialOutput=0
  wires:
  Clock/1 -> Sum1/1, Memory1/1
  Memory1/1 -> Sum1/2
  Sum1/1 -> out_1/1

== system lib_fuel_converter/fuel converter  <fc> for series/spinning up or spinning down/effect of inertia (Nm) ==
  note: if initial speed is >0 and it is the
      | first time step ignore inertial loads
      | tm:2/6/01
  req'd spd (rad/s) : Inport
  prev spd : Inport  Port=2
  Clock : Clock
  Constant : Constant  Value=fc_inertia
  Constant1 : Constant  Value=cyc_mph(1,2)
  Logical Operator : Logic  Operator=NAND
  Logical Operator1 : Logic  Operator=NOT
  Memory : Memory  X0=-0.1
  Memory1 : Memory
  Product1 : Product  Inputs=**/*  SaturateOnIntegerOverflow=on  RndMeth=Zero  InputSameDT=on  OutDataTypeStr=Inherit: Same as first input
  Sum : Sum  Inputs=+-  SaturateOnIntegerOverflow=on  InputSameDT=on  OutDataTypeStr=Inherit: Same as first input
  Sum1 : Sum  Inputs=+-  SaturateOnIntegerOverflow=on  InputSameDT=on  OutDataTypeStr=Inherit: Same as first input
  (Nm) : Outport  InitialOutput=0
  wires:
  Logical Operator1/1 -> Logical Operator/2
  Memory1/1 -> Logical Operator1/1
  Constant1/1 -> Logical Operator/1
  Logical Operator/1 -> Product1/4
  Sum/1 -> Product1/2
  Sum1/1 -> Product1/3
  req'd spd (rad/s)/1 -> Sum/1
  prev spd/1 -> Sum/2
  Product1/1 -> (Nm)/1
  Memory/1 -> Sum1/2
  Clock/1 -> Memory1/1, Memory/1, Sum1/1
  Constant/1 -> Product1/1

== system lib_fuel_converter/fuel converter  <fc> for series/spinning up or spinning down/just started spin-down/spin-up ==
  state : Inport
  Logical Operator : Logic
  Logical Operator1 : Logic  Operator=NOT  Inputs=1
  Memory1 : Memory  X0=(cyc_mph(1,2)==0)
  trigger : Outport  InitialOutput=0
  wires:
  Memory1/1 -> Logical Operator1/1
  Logical Operator1/1 -> Logical Operator/2
  Logical Operator/1 -> trigger/1
  state/1 -> Logical Operator/1, Memory1/1

== system lib_fuel_converter/fuel converter  <fc> for series/spinning up or spinning down/no-lag Reset Integrator ==
  in_1 : Inport
  in_2 : Inport  Port=2
  in_3 : Inport  Port=3
  Constant : Constant  Value=0
  Memory : Memory  X0=initval
  Product : Product  SaturateOnIntegerOverflow=on  RndMeth=Zero  InputSameDT=on  OutDataTypeStr=Inherit: Same as first input
  Sum : Sum  SaturateOnIntegerOverflow=on  InputSameDT=on  OutDataTypeStr=Inherit: Same as first input
  Switch : Switch  Threshold=eps  SaturateOnIntegerOverflow=on  InputSameDT=on
  dt : Subsystem
  in_2==0 : RelationalOperator  Operator===  InputSameDT=on
  out_1 : Outport  InitialOutput=0
  wires:
  in_3/1 -> Switch/3
  in_2/1 -> in_2==0/1
  in_1/1 -> Product/2
  dt/1(out_1) -> Product/1
  Product/1 -> Sum/2
  Memory/1 -> Sum/1
  Sum/1 -> Switch/1
  Switch/1 -> out_1/1, Memory/1
  in_2==0/1 -> Switch/2
  Constant/1 -> in_2==0/2
